simulink model "DC_motor_1_ode"  (R2022a)
settings: Solver=VariableStepAuto  StartTime=0.0  StopTime=10.0  RelTol=1e-3
settings Model: Creator=Adarsh  LastModifiedBy=Adarsh

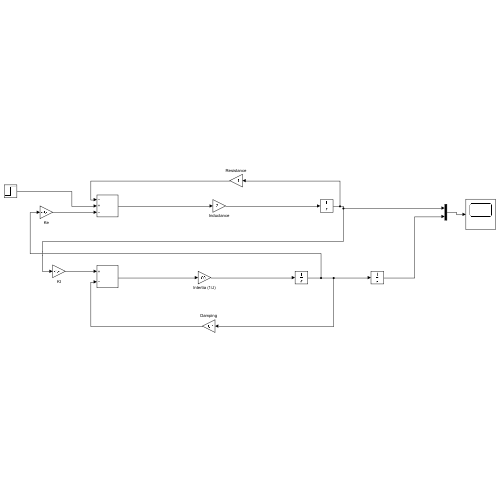
[thumbnail: Simulink's stored preview of the top-level diagram]
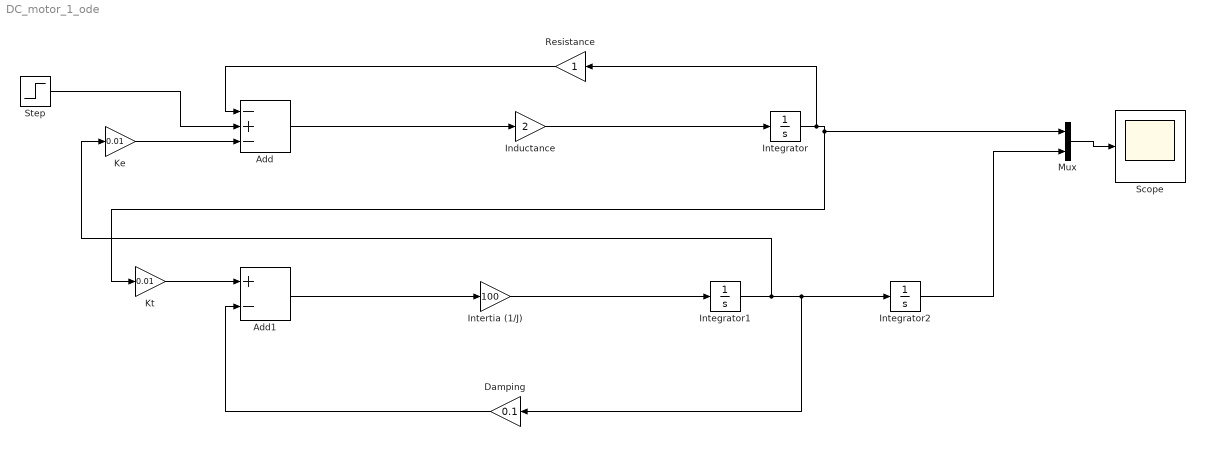
== system DC_motor_1_ode ==
  Add : Sum  Inputs=-+-
  Add1 : Sum  Inputs=+-
  Damping : Gain  Gain=0.1
  Inductance : Gain  Gain=2
  Integrator : Integrator
  Integrator1 : Integrator
  Integrator2 : Integrator
  Intertia (1/J) : Gain  Gain=100
  Ke : Gain  Gain=0.01
  Kt : Gain  Gain=0.01
  Mux : Mux  Inputs=2
  Resistance : Gain
  Scope : Scope
  Step : Step  SampleTime=0
  wires:
  Add/1 -> Inductance/1
  Inductance/1 -> Integrator/1
  Add1/1 -> Intertia (1/J)/1
  Intertia (1/J)/1 -> Integrator1/1
  Integrator/1 -> Resistance/1, Kt/1, Mux/1
  Kt/1 -> Add1/1
  Resistance/1 -> Add/1
  Integrator1/1 -> Ke/1, Damping/1, Integrator2/1
  Damping/1 -> Add1/2
  Ke/1 -> Add/3
  Mux/1 -> Scope/1
  Integrator2/1 -> Mux/2
  Step/1 -> Add/2
